simulink model "RC_Circuit_Simlation"  (R2022b)
settings: Solver=VariableStepAuto  StartTime=0.0  StopTime=10.0  MaxStep=1e-3  RelTol=1e-3
values from neighbouring files (symbols this model uses):
  C = 1e-6    (= 1e-06)    [RC_Circuit_Simlation_main.m]
  R = RValues(i)    [RC_Circuit_Simlation_main.m]
settings Model: Creator=Mo_7atem  LastModifiedBy=Mo_7atem

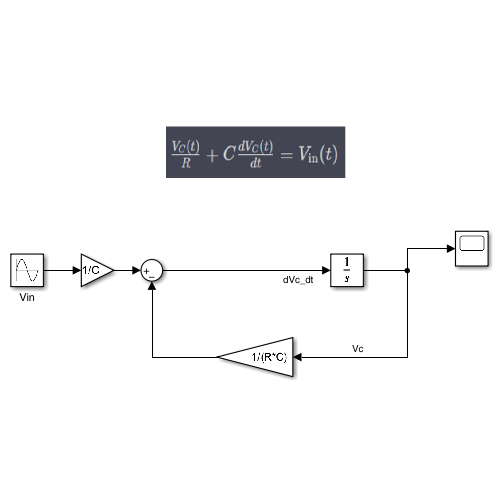
[thumbnail: Simulink's stored preview of the top-level diagram]
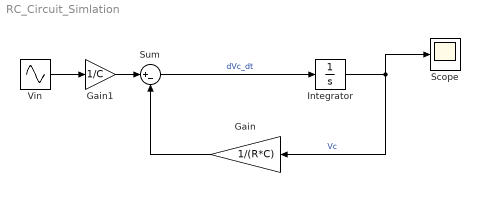
== system RC_Circuit_Simlation ==
  Gain : Gain  Gain=1/(R*C)
  Gain1 : Gain  Gain=1/C
  Integrator : Integrator
  Scope : Scope
  Sum : Sum  Inputs=|+-
  Vin : Sin  Amplitude=5  Frequency=2*pi  SampleTime=0
  wires:
  Vin/1 -> Gain1/1
  Integrator/1 -> Scope/1, Gain/1  "Vc"
  Sum/1 -> Integrator/1  "dVc_dt"
  Gain/1 -> Sum/2
  Gain1/1 -> Sum/1
